simulink model "control_diego"  (R2020b)
settings: Solver=VariableStepAuto  StartTime=0.0  StopTime=10  RelTol=1e-3
settings Model: Creator=Acer  LastModifiedBy=Acer

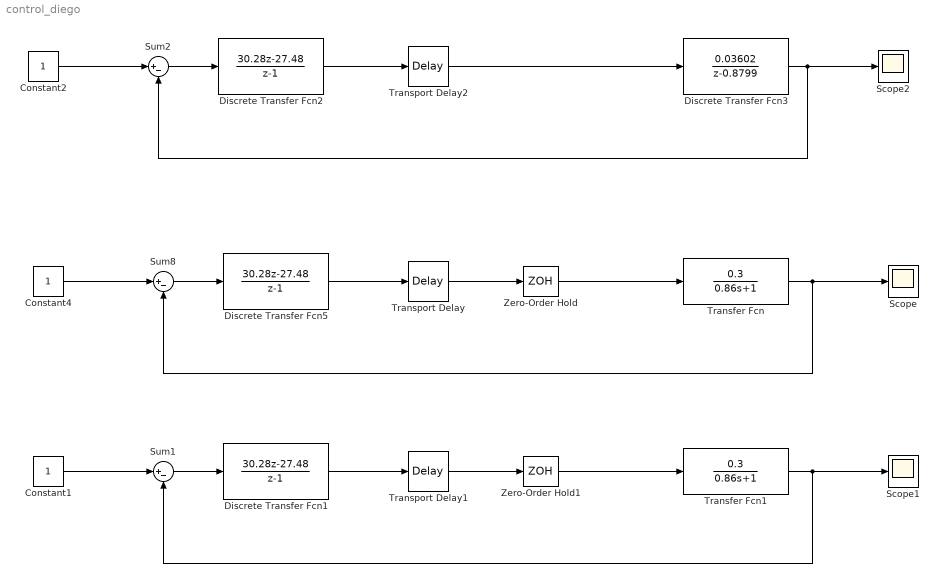
== system control_diego ==
  Constant1 : Constant
  Constant2 : Constant
  Constant4 : Constant
  Discrete Transfer Fcn1 : DiscreteTransferFcn  Numerator=[30.28 -27.48]  Denominator=[1 -1]  SampleTime=0.11
  Discrete Transfer Fcn2 : DiscreteTransferFcn  Numerator=[30.28 -27.48]  Denominator=[1 -1]  SampleTime=0.11
  Discrete Transfer Fcn3 : DiscreteTransferFcn  Numerator=0.03602  Denominator=[1 -0.8799]  SampleTime=0.11
  Discrete Transfer Fcn5 : DiscreteTransferFcn  Numerator=[30.28 -27.48]  Denominator=[1 -1]  SampleTime=0.11
  Scope : Scope
  Scope1 : Scope
  Scope2 : Scope
  Sum1 : Sum  Inputs=|+-
  Sum2 : Sum  Inputs=|+-
  Sum8 : Sum  Inputs=|+-
  Transfer Fcn : TransferFcn  Numerator=0.3  Denominator=[0.86 1]
  Transfer Fcn1 : TransferFcn  Numerator=0.3  Denominator=[0.86 1]
  Transport Delay : TransportDelay  DelayTime=0.00001
  Transport Delay1 : TransportDelay  DelayTime=0
  Transport Delay2 : TransportDelay  DelayTime=0
  Zero-Order Hold : ZeroOrderHold  SampleTime=0.11
  Zero-Order Hold1 : ZeroOrderHold  SampleTime=0.11
  wires:
  Sum8/1 -> Discrete Transfer Fcn5/1
  Constant4/1 -> Sum8/1
  Discrete Transfer Fcn5/1 -> Transport Delay/1
  Transport Delay/1 -> Zero-Order Hold/1
  Zero-Order Hold/1 -> Transfer Fcn/1
  Transfer Fcn/1 -> Scope/1, Sum8/2
  Transfer Fcn1/1 -> Scope1/1, Sum1/2
  Zero-Order Hold1/1 -> Transfer Fcn1/1
  Sum1/1 -> Discrete Transfer Fcn1/1
  Constant1/1 -> Sum1/1
  Transport Delay1/1 -> Zero-Order Hold1/1
  Discrete Transfer Fcn1/1 -> Transport Delay1/1
  Discrete Transfer Fcn3/1 -> Scope2/1, Sum2/2
  Discrete Transfer Fcn2/1 -> Transport Delay2/1
  Sum2/1 -> Discrete Transfer Fcn2/1
  Constant2/1 -> Sum2/1
  Transport Delay2/1 -> Discrete Transfer Fcn3/1
